simulink model "CM13_2024a_MachE_for_UA_HIL"  (R2024a)
settings: Solver=ode1  StartTime=0.0  StopTime=Inf  FixedStep=0.001  RelTol=1e-3  EnableMultiTasking=on
PreLoadFcn:
  | % if ~length(which('cmcmd')), cmenv; end
PostLoadFcn:
  | if any(exist('dsrtsu_mdlpostloadfcn', 'file') ~= 0), dsrtsu_mdlpostloadfcn('Execute', bdroot); end
InitFcn:
  | , if any(exist('rtifpga_mdlclblib', 'file') ~= 0), rtifpga_mdlclblib('Init', bdroot); end,
  | , if any(exist('dsmpb_private', 'file') ~= 0), dsmpb_private('dsmpb_mdlclblib', 'Init', bdroot); end,
values from neighbouring files (symbols this model uses):
  CoastDown =     [Run_Simulink.mat]
  limitedMCT =     [Run_Simulink.mat]
  MCT =     [Run_Simulink.mat]
  pMCT =     [Run_Simulink.mat]
  RealSimPara =     [Run_Simulink.mat]
  Ref_speed = [13 13.007895099 13.015778396 13.023649891 13.031509584 13.039357475 13.047193564 13.055017851 13.062830336 13.070631019 13.0784199 13.086196979 ... (2669 elements, 2669x1)]    [Ref_speed_and_time.mat]
  Ref_time = [0 0.01 0.02 0.03 0.04 0.05 0.06 0.07 0.08 0.09 0.1 0.11 ... (2669 elements, 2669x1)]    [Ref_speed_and_time.mat]
  US06 =     [Run_Simulink.mat]
undefined symbols (not defined in the file or in its folder): AccelCmd, ActTqLF_Nm_, ActTqLR_Nm_, ActTqRF_Nm_, ActTqRR_Nm_, BattChargeLimitMaxPwr, BattChargeLimitSocBpts, BattChargeLimitTbl, BattChrgCapcty, BattDischargeLimitSocBpts, BattDischargeLimitTbl, BattDischargeMaxPwr, BattNumCellsParallel, BattNumCellsSeries, BattOpenVoltCapBpts, BattOpenVoltTbl, BattResistSocBpts, BattResistTbl, BattResistTempBpts, BrakeMaxPrs, BrakeMaxTrq, ChassisDistCg2FrontAxle, ChassisDistCg2RearAxle, ChassisVehMass, CltchCmd, DecelCmd, DiffRatio, DiscIntNeverNeededParam, EnvGravCnst, EnvPrs, EnvTemp, FuelSpecificGrav, GearCmd, h, InitStates, lgSw, MtrEffSpdBpts, MtrEffTbl, MtrEffTrqBpts, MtrPwrMax, MtrTrqMax, planned_speed, planned_time, ref_speed, ref_time, rticanmm_blockfcn, rticanmm_initfcn, SteeringCmd, SupvsryCtrlRegenBrkCutOffTbl, SupvsryCtrlRegenSpdBpts, TestScnrioCycleNum, VEH
libraries: simulink x264, VSIGenLib x262, etargetslib x201, dsmpblib x161, CarMaker4SL x142, rtimmsu_dsrtlib x32, vehdynlibtire x24, autolibshared x19, vehdynlibsuspension x14, vehdynlibtirecommon x14, autolibutils x10, VsrLibWheel x8
(part 6 of 48)

== system CM13_2024a_MachE_for_UA_HIL/CarMaker/IPG Vehicle/Driver and Drive Cycle ==
  note: Rate Limiter note:
      | wet ground test: 7, -9.8
      | Ford default 5, -5
  note: Traffic light index:
      | Scenario based hack
      | 4,190,316 for UA road, route:Left lane straite
  note: Traffic light state/phase (integer):
      | 0: All lights off
      | 1: Green light on
      | 2: Yellow light on
      | 3: Red light on
      | 4: Red-Yellow light on
  note: Camera object type (integer)
      | 0 - Car
      | 1 - Truck
      | 2 - Bicycle
      | 3 - Pedestrian
      | 4 - Traffic sign
      | 5 - Traffic light
  note: DriveCycle temp comment out
  note: This selector in ControlDesk:
      | BYPASS CONTROLS -> ManSpdSel
      | Manual input in km/h
      | #Temp disabledl, 0 Speed
      | Speed from a IDM
      | Read from CM testrun file (this is for CRADA project automation)
      | 5. Speed from eco-driving history
      | 6. Zero speed
  Veh speed feedback [kph] : Inport
  Veh speed cycle trigger : Inport  Port=2
  AEB_IS_Triggered : Inport  Port=3
  "Auto_M_SW_Sig " : Inport  Port=4
  SUMO_spd : Inport  Port=5
  CM_Time : Inport  Port=6
  VehSpdRef : Inport  Port=7
  Add : Sum
  Add1 : Sum  Commented=on  Inputs=+-
  Add2 : Sum  Commented=on
  Add3 : Sum  Commented=on  Inputs=+-
  Automation_Spd_selection : Subsystem  Commented=on
  Automation_spd : Terminator
  Automation_spd1 : Terminator
  Bus Selector2 : BusSelector  Commented=on  OutputSignals=ObjID,Type,LightState
  CM state : Scope  Commented=on
  CM_drv_act_kmh : Scope  Commented=on
  Cam_obj_index : Constant  Commented=on  Value=0
  Camera Sensor Object : CarMaker4SL/Sensors/Camera Sensor Object  Commented=on  xname=1  xstime=Continuous
      settings: SourceProductName=CarMaker4SL
  CarV_kmh : Scope  Commented=on
  CaraX_ ms2 : Scope  Commented=on
  Clock{1..4} (4 alike) : Clock  Commented=on
  CoastDown : Lookup_n-D  Commented=through  NumberOfTableDimensions=1  BreakpointsForDimension1=CoastDown.Time  Table=CoastDown.Speed  InternalRulePriority=Speed  RndMeth=Simplest
  Compare To Constant : simulink/Logic and Bit Operations/Compare To Constant  Commented=on  relop===  const=8  OutDataTypeStr=boolean
  Constant : Constant  Value=6
  Constant1 : Constant  Value=0
  Constant2 : Constant  Value=5
  Constant3 : Constant  Value=0
  Constant4 : Constant  Commented=on  Value=0
  Data Type Conversion11 : DataTypeConversion  OutDataTypeStr=double  SaturateOnIntegerOverflow=off  RndMeth=Floor  LockScale=on
  Dis2lead_IPGdriver : Scope  Commented=on
  DriveCycleSelect : Constant
  Driver and PI with FF Control : Subsystem
  From4 : From  Commented=on  GotoTag=VehSpdRef  TagVisibility=global
  Gain : Gain  Gain=1/1.609
  Gain1 : Gain  Gain=1/1.609
  Gain2 : Gain  Gain=3.6
  Gain3 : Gain  Gain=3.6
  Gain4 : Gain  Commented=on  Gain=3.6
  Gain5 : Gain  Commented=on  Gain=3.6
  Gain6 : Gain  Commented=on  Gain=1.609
  Gain7 : Gain  Commented=on  Gain=1.609
  Get Cycle Clock Time : Subsystem  Commented=through
  IDM : Subsystem  Commented=on
  IDM Rate Limiter : RateLimiter  RisingSlewLimit=1.2  FallingSlewLimit=-6.5  SampleTimeMode=inherited
  Jinghui planned speed : Lookup_n-D  Commented=on  NumberOfTableDimensions=1  BreakpointsForDimension1=planned_time  Table=planned_speed  InternalRulePriority=Speed  RndMeth=Simplest
  LightState : Scope  Commented=on
  MCT : Lookup_n-D  Commented=through  NumberOfTableDimensions=1  BreakpointsForDimension1=MCT.Time  Table=MCT.Speed  InternalRulePriority=Speed  RndMeth=Simplest
  ManSpd : Constant  Value=0
  ManSpdSel : Constant
  Maxkmh_limiter : Saturate  UpperLimit=120  LowerLimit=0
  Memory1 : Memory  Commented=on
  Memory2 : Memory  Commented=on
  Minus : Sum  Commented=on  Inputs=+-
  Minus1 : Sum  Commented=on  Inputs=+-
  Multiport Switch : MultiPortSwitch  Inputs=5  SaturateOnIntegerOverflow=off  InputSameDT=off
  Multiport Switch1 : MultiPortSwitch  Inputs=7  SaturateOnIntegerOverflow=off  InputSameDT=off
  ObjectIndex : Scope  Commented=on
  Rate Limiter : RateLimiter  RisingSlewLimit=5  FallingSlewLimit=-5  SampleTimeMode=inherited
  Rate Limiter1 : RateLimiter  RisingSlewLimit=5  FallingSlewLimit=-5  SampleTimeMode=inherited
  Read CM Dict : CarMaker4SL/Read CM Dict  Commented=on  xname=SC.State  xsync=off  xstime=Continuous
  Read CM Dict1 : CarMaker4SL/Read CM Dict  Commented=on  xname=Car.ax  xsync=off  xstime=Continuous
  Read CM Dict2 : CarMaker4SL/Read CM Dict  Commented=on  xname=Driver.ReCon.Speed  xsync=off  xstime=Continuous
  Read CM Dict3 : CarMaker4SL/Read CM Dict  Commented=on  xname=Driver.Long.dv  xsync=off  xstime=Continuous
  Read CM Dict4 : CarMaker4SL/Read CM Dict  Commented=on  xname=Driver.ReCon.Trf_FOL.dDist  xsync=off  xstime=Continuous
  Read CM Dict5 : CarMaker4SL/Read CM Dict  Commented=on  xname=Car.v  xsync=off  xstime=Continuous
  Switch : Switch  Commented=on  Criteria=u2 ~= 0  SaturateOnIntegerOverflow=off  InputSameDT=off
  Switch1 : Switch  Commented=on  SaturateOnIntegerOverflow=off  InputSameDT=off
  Switch2 : Switch  Commented=on  SaturateOnIntegerOverflow=off  InputSameDT=off
  Terminator : Terminator
  Terminator1 : Terminator
  Terminator2 : Terminator  Commented=on
  Terminator3 : Terminator  Commented=on
  Terminator4 : Terminator
  US06 : Lookup_n-D  Commented=through  NumberOfTableDimensions=1  BreakpointsForDimension1=US06.Time  Table=US06.Speed  InternalRulePriority=Speed  RndMeth=Simplest
  driver look ahead seconds : Constant  Value=0.5
  limitedMCT : Lookup_n-D  Commented=through  NumberOfTableDimensions=1  BreakpointsForDimension1=limitedMCT.Time  Table=limitedMCT.Speed  InternalRulePriority=Speed  RndMeth=Simplest
  pMCT : Lookup_n-D  Commented=through  NumberOfTableDimensions=1  BreakpointsForDimension1=pMCT.Time  Table=pMCT.Speed  InternalRulePriority=Speed  RndMeth=Simplest
  real veh speed : Lookup_n-D  Commented=on  NumberOfTableDimensions=1  BreakpointsForDimension1=ref_time  Table=ref_speed  InternalRulePriority=Speed  RndMeth=Simplest
  DriverBus : Outport
  wires:
  Veh speed cycle trigger/1 -> Get Cycle Clock Time/1(Cycle Trigger)
  MCT/1 -> Multiport Switch/5
  US06/1 -> Multiport Switch/4
  Add/1 -> CoastDown/1, pMCT/1, limitedMCT/1, MCT/1, US06/1
  CoastDown/1 -> Multiport Switch/2
  pMCT/1 -> Multiport Switch/3
  DriveCycleSelect/1 -> Multiport Switch/1
  [VehSpdKph] -> Data Type Conversion11/1
  Driver and PI with FF Control/1(DriverBus) -> DriverBus/1
  Data Type Conversion11/1 -> Gain/1, Driver and PI with FF Control/1(Vehicle_Spd_kph)  "Vehicle_Spd_kph"
  Get Cycle Clock Time/1(tCycle) -> Add/2
  driver look ahead seconds/1 -> Add/1
  limitedMCT/1 -> Multiport Switch/6
  Veh speed feedback [kph]/1 -> [VehSpdKph]
  Gain/1 -> Terminator/1  "Vehicle_Spd_mph"
  Gain1/1 -> Terminator1/1  "Vehicle_SpdDmd_mph"
  ManSpd/1 -> Rate Limiter/1
  Rate Limiter/1 -> Multiport Switch1/2
  Multiport Switch/1 -> Automation_spd1/1
  Constant1/1 -> Multiport Switch1/8
  Automation_Spd_selection/1(Spd) -> Rate Limiter1/1, Automation_spd/1  "Automation_spd"
  AEB_IS_Triggered/1 -> Automation_Spd_selection/1(AEB_IS_Triggered)
  "Auto_M_SW_Sig "/1 -> Automation_Spd_selection/2(A_M_SW_sig)
  Rate Limiter1/1 -> Multiport Switch1/5
  SUMO_spd/1 -> Terminator4/1
  Gain2/1 -> Multiport Switch1/3  "Vehicle_SpdDmd_kmh"
  Read CM Dict4/1 -> Dis2lead_IPGdriver/1  "Trf_FOL_dDist"
  Gain3/1 -> Maxkmh_limiter/1  "Vehicle_SpdDmd_kmh"
  Maxkmh_limiter/1 -> Multiport Switch1/4
  Read CM Dict2/1 -> Add2/1
  Read CM Dict3/1 -> Gain4/1
  Gain4/1 -> Add2/2
  Read CM Dict5/1 -> Gain5/1  "VehSpd"
  Gain5/1 -> CarV_kmh/1
  Add2/1 -> CM_drv_act_kmh/1
  Camera Sensor Object/2 -> Bus Selector2/1
  Bus Selector2/1 -> Terminator2/1  "<ObjID>"
  Bus Selector2/2 -> Terminator3/1  "<Type>"
  Bus Selector2/3 -> LightState/1  "<LightState>"
  Cam_obj_index/1 -> Camera Sensor Object/2
  Camera Sensor Object/1 -> ObjectIndex/1
  Read CM Dict1/1 -> CaraX_ ms2/1  "VehSpd"
  CM_Time/1 -> IDM/1(CM_Time)
  Clock3/1 -> Add1/1
  ManSpdSel/1 -> Minus/1, Minus1/1, Multiport Switch1/1
  real veh speed/1 -> Gain6/1
  Clock2/1 -> Switch2/3
  Memory1/1 -> Switch2/1
  Add1/1 -> real veh speed/1  "tCycle"
  Switch2/1 -> Add1/2, Memory1/1
  Gain6/1 -> Multiport Switch1/6  "realV"
  Clock1/1 -> Switch1/3
  Add3/1 -> Jinghui planned speed/1  "tCycle"
  Memory2/1 -> Switch1/1
  Switch1/1 -> Add3/2, Memory2/1
  Clock4/1 -> Add3/1
  Jinghui planned speed/1 -> Gain7/1
  Gain7/1 -> Multiport Switch1/7  "refV"
  Constant/1 -> Minus/2
  Minus/1 -> Switch1/2
  Constant2/1 -> Minus1/2
  Minus1/1 -> Switch2/2
  Constant3/1 -> Gain2/1
  Multiport Switch1/1 -> Gain1/1, Driver and PI with FF Control/2(Vehicle_SpdDmd_kph)  "RefSpd [km/hr]"
  Read CM Dict/1 -> CM state/1, Compare To Constant/1
  Constant4/1 -> Switch/3
  Compare To Constant/1 -> Switch/2
  IDM Rate Limiter/1 -> Gain3/1
  VehSpdRef/1 -> IDM Rate Limiter/1

== system CM13_2024a_MachE_for_UA_HIL/CarMaker/IPG Vehicle/FD1 ==
  Bus Selector : BusSelector  OutputSignals=Simulated ECUs.FD1_CAN_P702_BEV_MY22_DCV_v12_06-7-2021.FD1_CAN_HCM.RX.PDUs.Body_Info_10_FD1.PosLghtFr_D_Stat.ISignal Value.GearRvrse_D_Actl Value,Simulated ECUs.FD1_CAN_P702_BEV_MY22_DCV_v12_06-7-2021.FD1_CAN_HCM.RX.PDUs.PowertrainData_10.TrnRng_D_Rq.ISignal Value.TrnRng_D_Rq Value,Simulated ECUs.FD1_CAN_P702_BEV_MY22_DCV_v12_06-7-2021.FD1_CAN_HCM.RX.PDUs.PowertrainData_10.TrnPrkSys_D_Actl.ISignal Value.TrnPrkSys_D_Actl Value,Simulated ECUs.FD1_CAN_P702_BEV_MY22_DCV_v12_06-7-2021.FD1_CAN_HCM.RX.PDUs.PowertrainData_10.GearLvr_D_ActlDrv.ISignal Value.GearLvr_D_ActlDrv Value,Simulated ECUs.FD1_CAN_P702_BEV_MY22_DCV_v12_06-7-2021.FD1_CAN_HCM.RX.PDUs.PowertrainData_10.GearPos_D_Actl.ISignal Value.GearPos_D_Actl Value
  MachE_CANConfig_In : dsmpblib/Data Inport  Priority=10000
      settings: SourceProductName=dSPACE Model Interface Package for Simulink (MIPS)
  Terminator{,8..9,14..15} (5 alike) : Terminator
  wires:
  Bus Selector/2 -> Terminator8/1  "<TrnRng_D_Rq Value>"
  MachE_CANConfig_In/1 -> Bus Selector/1
  Bus Selector/1 -> Terminator/1  "<GearRvrse_D_Actl Value>"
  Bus Selector/3 -> Terminator9/1  "<TrnPrkSys_D_Actl Value>"
  Bus Selector/5 -> Terminator15/1  "<GearPos_D_Actl Value>"
  Bus Selector/4 -> Terminator14/1  "<GearLvr_D_ActlDrv Value>"

== system CM13_2024a_MachE_for_UA_HIL/CarMaker/IPG Vehicle/From CAN ==
  Steering_ang_deg : Inport
  BrakeSwitch : Inport  Port=2
  Brake switch ource selection : Constant  Value=2
  Bus Creator1 : BusCreator  Inputs=2
  Demux : Demux  Outputs=1
  Ground1 : Ground
  Multiport Switch1 : MultiPortSwitch  Inputs=2  SaturateOnIntegerOverflow=off  InputSameDT=off
  IO_Out : Outport
  wires:
  Bus Creator1/1 -> IO_Out/1  "IO_Out"
  Multiport Switch1/1 -> Bus Creator1/2  "BRAKE_LAMP_BOOL_CAN"
  Demux/1 -> Bus Creator1/1  "STEERING_ANGLE_DEG_CAN"
  Steering_ang_deg/1 -> Demux/1
  Brake switch ource selection/1 -> Multiport Switch1/1
  Ground1/1 -> Multiport Switch1/2  "Brake switch from CAN"
  BrakeSwitch/1 -> Multiport Switch1/3

== system CM13_2024a_MachE_for_UA_HIL/CarMaker/IPG Vehicle/Mach-E CAN BM ==
  note: Reading energy from MachE battery
  Add : Sum
  Bus Creator : BusCreator  Inputs=3
  Bus Creator1 : BusCreator  Inputs=5
  Bus Creator2 : BusCreator  Inputs=5
  Bus Selector : BusSelector  OutputSignals=Simulated ECUs.HS2_2022MY_P702_FNV2_BEV_DCV_v35.GWM.RX.PDUs.Yaw_Data.VehRol_W_Actl.ISignal Value.VehRol_W_Actl Value,Simulated ECUs.HS2_2022MY_P702_FNV2_BEV_DCV_v35.GWM.RX.PDUs.Yaw_Data.VehYaw_W_Actl.ISignal Value.VehYaw_W_Actl Value,Simulated ECUs.HS2_2022MY_P702_FNV2_BEV_DCV_v35.OCS.RX.PDUs.Accel_Data.VehLong2_A_Actl.ISignal Value.VehLong2_A_Actl Value,Simulated ECUs.HS2_2022MY_P702_FNV2_BEV_DCV_v35.OCS.RX.PDUs.Accel_Data.VehLat2_A_Actl.ISignal Value.VehLat2_A_Actl Value,Simulated ECUs.HS2_2022MY_P702_FNV2_BEV_DCV_v35.OCS.RX.PDUs.Accel_Data.VehVert2_A_Actl.ISignal Value.VehVert2_A_Actl Value
  Bus Selector1 : BusSelector  OutputSignals=Simulated ECUs.HS2_2022MY_P702_FNV2_BEV_DCV_v35.RCM.RX.PDUs.SteeringPinion_Data_HS2.StePinRelInit_An_Sns.ISignal Value.StePinRelInit_An_Sns Value
  Bus Selector2 : BusSelector  Commented=on  OutputSignals=VehRol_W_Actl Value,VehYaw_W_Actl Value,VehLong2_A_Actl Value,VehLat2_A_Actl Value,VehVert2_A_Actl Value
  Bus Selector3 : BusSelector  OutputSignals=Simulated ECUs.HS1_CAN_P702_BEV_MY22_DCV_v12_06-7-2021.GWM.RX.PDUs.Battery_Traction_2.BattTrac_U2_Actl.ISignal Value.BattTrac_U2_Actl Value,Simulated ECUs.HS1_CAN_P702_BEV_MY22_DCV_v12_06-7-2021.GWM.RX.PDUs.Battery_Traction_2.BattTrac_I2_Actl.ISignal Value.BattTrac_I2_Actl Value,Simulated ECUs.HS1_CAN_P702_BEV_MY22_DCV_v12_06-7-2021.GWM.RX.PDUs.Battery_Traction_9.BattChrg_I2_Rq.ISignal Value.BattChrg_I2_Rq Value,Simulated ECUs.HS1_CAN_P702_BEV_MY22_DCV_v12_06-7-2021.GWM.RX.PDUs.Battery_Traction_9.BattChrg_I2_Mx.ISignal Value.BattChrg_I2_Mx Value,Simulated ECUs.HS1_CAN_P702_BEV_MY22_DCV_v12_06-7-2021.GWM.RX.PDUs.Battery_Traction_7.BattChrg_U_Mx.ISignal Value.BattChrg_U_Mx Value,Simulated ECUs.HS1_CAN_P702_BEV_MY22_DCV_v12_06-7-2021.GWM.RX.PDUs.DataMonitoring_2.Mtr4Aout_Tq_ActlMntr.ISignal Value.Mtr4Aout_Tq_ActlMntr Value,Simulated ECUs.HS1_CAN_P702_BEV_MY22_DCV_v12_06-7-2021.GWM.RX.PDUs.DataMonitoring_2.Mtr4Aout_W_ActlMntr.ISignal Value.Mtr4Aout_W_ActlMntr Value,Simulated ECUs.HS1_CAN_P702_BEV_MY22_DCV_v12_06-7-2021.SOBDMB_AWDC.RX.PDUs.EngVehicleSpThrottle_HS1.EngAout3_N_Actl.ISignal Value.EngAout3_N_Actl Value,Simulated ECUs.HS1_CAN_P702_BEV_MY22_DCV_v12_06-7-2021.SOBDMB_AWDC.RX.PDUs.EngVehicleSpThrottle_HS1.EngAout_N_Actl.ISignal Value.EngAout_N_Actl Value,Simulated ECUs.HS1_CAN_P702_BEV_MY22_DCV_v12_06-7-2021.SOBDM_BCCM.RX.PDUs.EngineClimateData_HS1.EngAout_Aa_Actl.ISignal Value.EngAout_Aa_Actl Value,Simulated ECUs.HS1_CAN_P702_BEV_MY22_DCV_v12_06-7-2021.BCM.RX.PDUs.EngineData_6_HS1.EngGoutLss_Tq_Est.ISignal Value.EngGoutLss_Tq_Est Value
  Cast : DataTypeConversion  OutDataTypeStr=uint32  SaturateOnIntegerOverflow=off  RndMeth=Floor
  Cast To Boolean : DataTypeConversion  OutDataTypeStr=boolean  SaturateOnIntegerOverflow=off  RndMeth=Floor
  Cast To Boolean1 : DataTypeConversion  OutDataTypeStr=boolean  SaturateOnIntegerOverflow=off  RndMeth=Floor
  Constant : Constant
  Constant1 : Constant
  Constant2 : Constant  Value=3
  Demux : Demux  Outputs=5
  Harness_Cfg_Out : dsmpblib/Data Outport  Priority=-10000
      settings: SourceProductName=dSPACE Model Interface Package for Simulink (MIPS)
  MachE_HS1_Config_In : dsmpblib/Data Inport  Priority=10000
      settings: SourceProductName=dSPACE Model Interface Package for Simulink (MIPS)
  RCM Pass-Through : Constant
  RCM_Cfg_In : dsmpblib/Data Inport  Priority=10000
      settings: SourceProductName=dSPACE Model Interface Package for Simulink (MIPS)
  RCM_Cfg_Out (1) : dsmpblib/Data Outport  Priority=-10000
      settings: SourceProductName=dSPACE Model Interface Package for Simulink (MIPS)
  Steering Sensor Offset : Constant  Value=0
  Subsystem : Subsystem  Commented=on
  Subsystem1 : Subsystem  Commented=on
  Switch : Switch  Criteria=u2 > Threshold  SaturateOnIntegerOverflow=off  InputSameDT=off
  Terminator{,1..10} (11 alike) : Terminator
  Steering_Out : Outport
  wires:
  Constant/1 -> Cast To Boolean/1
  Constant1/1 -> Cast To Boolean1/1
  Constant2/1 -> Cast/1
  Cast/1 -> Bus Creator/3  "Frame Gateway (1) Direction"
  Cast To Boolean/1 -> Bus Creator/1  "CAN Cluster 1 Filter Enable"
  Cast To Boolean1/1 -> Bus Creator/2  "CAN Cluster 2 Filter Enable"
  MachE_HS1_Config_In/1 -> Bus Selector3/1
  Bus Creator/1 -> RCM_Cfg_Out (1)/1
  Demux/1 -> Bus Creator1/1  "VehRol_W_Actl Value"
  Demux/2 -> Bus Creator1/2  "VehYaw_W_Actl Value"
  Demux/3 -> Bus Creator1/3  "VehLong2_A_Actl Value"
  Demux/4 -> Bus Creator1/4  "VehLat2_A_Actl Value"
  Demux/5 -> Bus Creator1/5  "VehVert2_A_Actl Value"
  RCM_Cfg_In/1 -> Bus Selector/1, Bus Selector1/1
  RCM Pass-Through/1 -> Switch/2
  Subsystem/1(AccelYaw_out) -> Switch/3
  Switch/1 -> Demux/1
  Bus Selector/5 -> Bus Creator2/5  "<VehVert2_A_Actl Value>"
  Bus Selector/2 -> Bus Creator2/2  "<VehYaw_W_Actl Value>"
  Bus Selector/1 -> Bus Creator2/1  "<VehRol_W_Actl Value>"
  Bus Creator2/1 -> Switch/1, Bus Selector2/1
  Bus Selector/3 -> Bus Creator2/3  "<VehLong2_A_Actl Value>"
  Bus Selector/4 -> Bus Creator2/4  "<VehLat2_A_Actl Value>"
  Bus Creator1/1 -> Harness_Cfg_Out/1
  Bus Selector1/1 -> Add/1  "<StePinRelInit_An_Sns Value>"
  Steering Sensor Offset/1 -> Add/2
  Add/1 -> Steering_Out/1
  Bus Selector3/1 -> Terminator/1  "<BattTrac_U2_Actl Value>"
  Bus Selector3/2 -> Terminator1/1  "<BattTrac_I2_Actl Value>"
  Bus Selector3/3 -> Terminator2/1  "<BattChrg_I2_Rq Value>"
  Bus Selector3/4 -> Terminator3/1  "<BattChrg_I2_Mx Value>"
  Bus Selector3/5 -> Terminator4/1  "<BattChrg_U_Mx Value>"
  Bus Selector3/6 -> Terminator5/1  "<Mtr4Aout_Tq_ActlMntr Value>"
  Bus Selector3/7 -> Terminator6/1  "<Mtr4Aout_W_ActlMntr Value>"
  Bus Selector3/8 -> Terminator7/1  "<EngAout3_N_Actl Value>"
  Bus Selector3/9 -> Terminator8/1  "<EngAout_N_Actl Value>"
  Bus Selector3/10 -> Terminator9/1  "<EngAout_Aa_Actl Value>"
  Bus Selector3/11 -> Terminator10/1  "<EngGoutLss_Tq_Est Value>"
